simulink model "motorModel"  (R2024a)
settings: Solver=VariableStepAuto  StartTime=0.0  StopTime=20  RelTol=1e-3
settings Model: Creator=janho  LastModifiedBy=janho

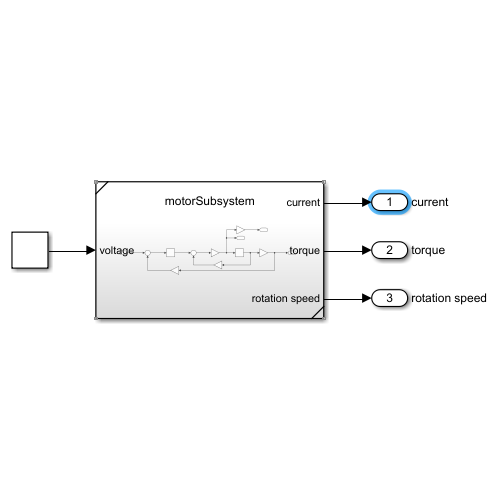
[thumbnail: Simulink's stored preview of the top-level diagram]
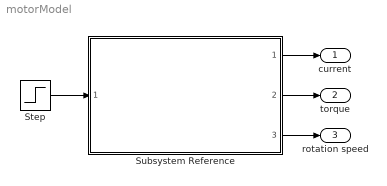
== system motorModel ==
  Step : Step  Time=0  After=10  SampleTime=0
  Subsystem Reference : Subsystem  ReferencedSubsystem=motorSubsystem
  current : Outport  SignalName=current
  torque : Outport  Port=2  SignalName=torque
  rotation speed : Outport  Port=3  SignalName=rotation speed
  wires:
  Subsystem Reference/2 -> torque/1
  Subsystem Reference/1 -> current/1
  Subsystem Reference/3 -> rotation speed/1
  Step/1 -> Subsystem Reference/1
